simulink model "DinamicaCinematicaControleAtitude"  (R2024a)
settings: Solver=FixedStepAuto  StartTime=0.0  StopTime=tf  FixedStep=step_modelo  RelTol=1e-3
values from neighbouring files (symbols this model uses):
  mi = 3.9860044189*10^14    (= 398600441890000)    [constantes.m]
undefined symbols (not defined in the file or in its folder): a0_ini, AttKd_x, AttKd_y, AttKd_z, AttKp_x, AttKp_y, AttKp_z, e0_ini, f0_ini, giro, giro_bias, giro_ruido, Ixx, Iyy, Izz, omega0_ini, omega1_rel_ini, omega2_rel_ini, omega3_rel_ini, phi_i, psi_i, theta_i
libraries: dspsrcs4 x3, matrix_library x2, sharedutil x2, aerolibutil x1
settings Model: Creator=rodri  LastModifiedBy=rodri
settings DataIOCC: SaveOutput=off  SaveTime=off
settings RTWCC: GPUComputeCapability=3.5

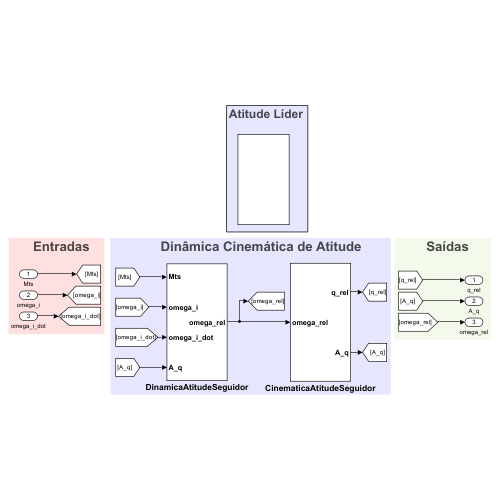
[thumbnail: Simulink's stored preview of the top-level diagram]
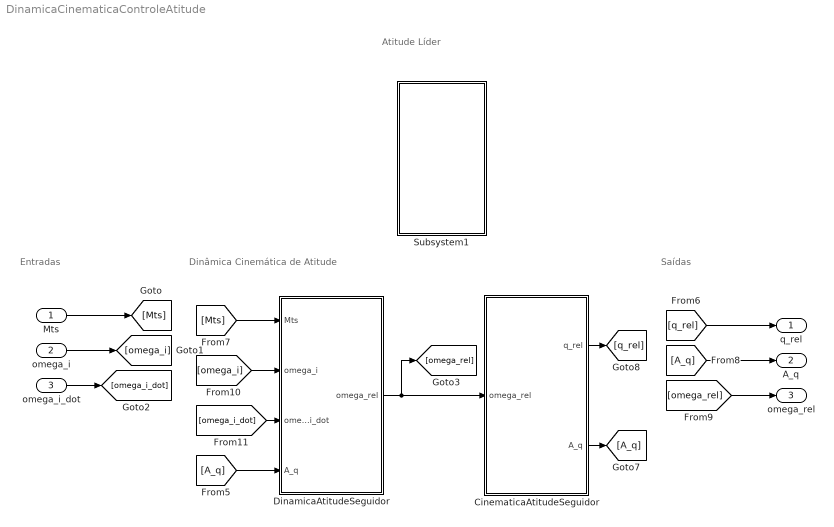
== system DinamicaCinematicaControleAtitude ==
  note: Dinâmica Cinemática de Atitude
  note: Entradas
  note: Saídas
  note: Atitude Líder
  Mts : Inport  OutDataTypeStr=double  PortDimensions=[3,1]
  omega_i : Inport  Port=2  OutDataTypeStr=double
  omega_i_dot : Inport  Port=3  OutDataTypeStr=double  PortDimensions=[3,1]
  CinematicaAtitudeSeguidor : Subsystem
  DinamicaAtitudeSeguidor : Subsystem
  Subsystem1 : Subsystem
  q_rel : Outport
  A_q : Outport  Port=2  PortDimensions=[3,3]
  omega_rel : Outport  Port=3
  wires:
  DinamicaAtitudeSeguidor/1(omega_rel) -> [omega_rel], CinematicaAtitudeSeguidor/1(omega_rel)
  CinematicaAtitudeSeguidor/2(A_q) -> [A_q]
  CinematicaAtitudeSeguidor/1(q_rel) -> [q_rel]
  omega_i/1 -> [omega_i]
  omega_i_dot/1 -> [omega_i_dot]
  [A_q] -> DinamicaAtitudeSeguidor/4(A_q)
  [Mts] -> DinamicaAtitudeSeguidor/1(Mts)
  [omega_i] -> DinamicaAtitudeSeguidor/2(omega_i)
  [omega_i_dot] -> DinamicaAtitudeSeguidor/3(omega_i_dot)
  [q_rel] -> q_rel/1
  [A_q] -> A_q/1
  [omega_rel] -> omega_rel/1
  Mts/1 -> [Mts]

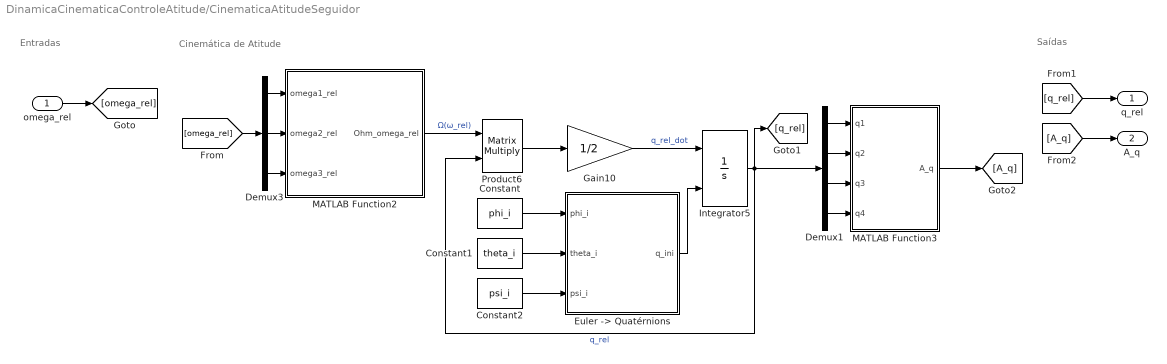
== system DinamicaCinematicaControleAtitude/CinematicaAtitudeSeguidor ==
  note: Cinemática de Atitude
  note: Entradas
  note: Saídas
  omega_rel : Inport
  Constant : Constant  Value=phi_i  SampleTime=-1
  Constant1 : Constant  Value=theta_i  SampleTime=-1
  Constant2 : Constant  Value=psi_i  SampleTime=-1
  Demux1 : Demux
  Demux3 : Demux  Outputs=3
  "Euler -> Quatérnions" : MATLAB Function  TreatAsAtomicUnit=on
  Gain10 : Gain  Gain=1/2
  Integrator5 : Integrator  InitialConditionSource=external  InitialCondition=[1; 0; 0; 0]
  MATLAB Function2 : MATLAB Function  TreatAsAtomicUnit=on
  MATLAB Function3 : MATLAB Function  TreatAsAtomicUnit=on
  Product6 : Product  Multiplication=Matrix(*)
  q_rel : Outport
  A_q : Outport  Port=2  PortDimensions=[3,3]
  wires:
  "Euler -> Quatérnions"/1(q_ini) -> Integrator5/2
  Demux1/2 -> MATLAB Function3/2(q2)
  Demux3/1 -> MATLAB Function2/1(omega1_rel)
  MATLAB Function2/1(Ohm_omega_rel) -> Product6/1  "Ω(ω_rel)"
  Demux1/4 -> MATLAB Function3/4(q4)
  Demux3/3 -> MATLAB Function2/3(omega3_rel)
  Demux3/2 -> MATLAB Function2/2(omega2_rel)
  Integrator5/1 -> Product6/2, Demux1/1, [q_rel]  "q_rel"
  Demux1/3 -> MATLAB Function3/3(q3)
  Gain10/1 -> Integrator5/1  "q_rel_dot"
  Demux1/1 -> MATLAB Function3/1(q1)
  Product6/1 -> Gain10/1
  [omega_rel] -> Demux3/1
  omega_rel/1 -> [omega_rel]
  [q_rel] -> q_rel/1
  [A_q] -> A_q/1
  MATLAB Function3/1(A_q) -> [A_q]
  Constant/1 -> "Euler -> Quatérnions"/1(phi_i)
  Constant1/1 -> "Euler -> Quatérnions"/2(theta_i)
  Constant2/1 -> "Euler -> Quatérnions"/3(psi_i)

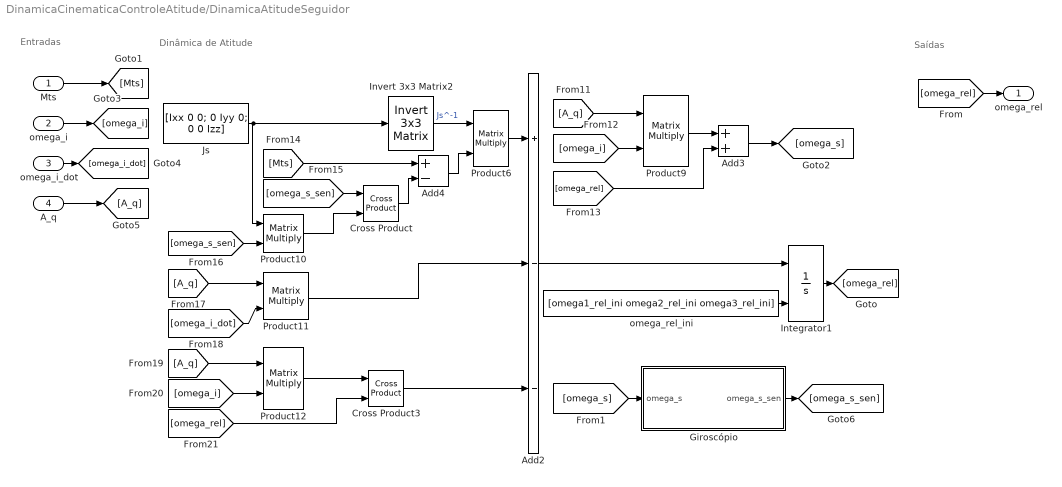
== system DinamicaCinematicaControleAtitude/DinamicaAtitudeSeguidor ==
  note: Dinâmica de Atitude
  note: Saídas
  note: Entradas
  Mts : Inport
  omega_i : Inport  Port=2
  omega_i_dot : Inport  Port=3
  A_q : Inport  Port=4
  Add2 : Sum  Inputs=+--
  Add3 : Sum
  Add4 : Sum  Inputs=+-
  Cross Product : matrix_library/Cross Product
  Cross Product3 : matrix_library/Cross Product
  Giroscópio : Subsystem
  Integrator1 : Integrator  InitialConditionSource=external  InitialCondition=[0; 0; 0]
  Invert 3x3 Matrix2 : aerolibutil/Invert  3x3 Matrix
  Js : Constant  Value=[Ixx 0 0; 0 Iyy 0; 0 0 Izz]
  Product{6,9..12} (5 alike) : Product  Multiplication=Matrix(*)
  omega_rel_ini : Constant  Value=[omega1_rel_ini omega2_rel_ini omega3_rel_ini]
  omega_rel : Outport
  wires:
  Integrator1/1 -> [omega_rel]
  Add2/1 -> Integrator1/1
  Invert 3x3 Matrix2/1 -> Product6/1  "Js^-1"
  omega_rel_ini/1 -> Integrator1/2
  [A_q] -> Product9/1
  [omega_i] -> Product9/2
  Product9/1 -> Add3/1
  [omega_rel] -> Add3/2
  Add3/1 -> [omega_s]
  [Mts] -> Add4/1
  Cross Product/1 -> Add4/2
  [omega_s_sen] -> Cross Product/1
  Js/1 -> Product10/1, Invert 3x3 Matrix2/1
  [omega_s_sen] -> Product10/2
  Product10/1 -> Cross Product/2
  Add4/1 -> Product6/2
  Product6/1 -> Add2/1
  [A_q] -> Product11/1
  [omega_i_dot] -> Product11/2
  Product11/1 -> Add2/2
  [A_q] -> Product12/1
  [omega_i] -> Product12/2
  Product12/1 -> Cross Product3/1
  [omega_rel] -> Cross Product3/2
  Cross Product3/1 -> Add2/3
  omega_i/1 -> [omega_i]
  A_q/1 -> [A_q]
  [omega_rel] -> omega_rel/1
  Mts/1 -> [Mts]
  omega_i_dot/1 -> [omega_i_dot]
  [omega_s] -> Giroscópio/1(omega_s)
  Giroscópio/1(omega_s_sen) -> [omega_s_sen]

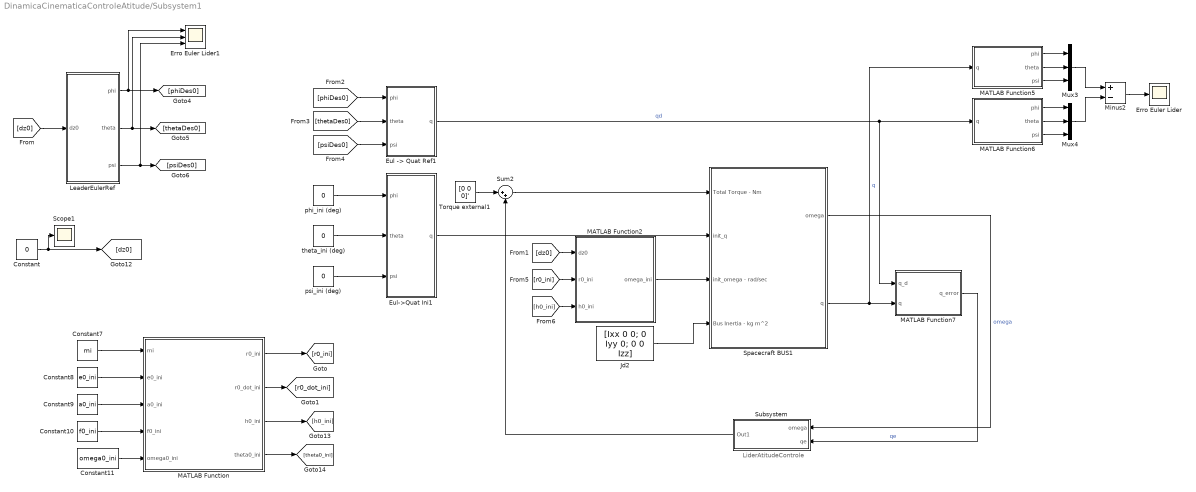
== system DinamicaCinematicaControleAtitude/Subsystem1 ==
  note: LiderAtitudeControle
  Constant : Constant  Value=0
  Constant10 : Constant  Value=f0_ini
  Constant11 : Constant  Value=omega0_ini
  Constant7 : Constant  Value=mi
  Constant8 : Constant  Value=e0_ini
  Constant9 : Constant  Value=a0_ini
  Erro Euler Lider : Scope
  Erro Euler Lider1 : Scope  NumInputPorts=3
  "Eul -> Quat Ref1" : MATLAB Function  TreatAsAtomicUnit=on
  Eul->Quat Ini1 : MATLAB Function  TreatAsAtomicUnit=on
  Jd2 : Constant  Value=[Ixx 0 0; 0 Iyy 0; 0 0 Izz]
  LeaderEulerRef : Subsystem
  MATLAB Function : MATLAB Function  TreatAsAtomicUnit=on
  MATLAB Function2 : MATLAB Function  TreatAsAtomicUnit=on
  MATLAB Function5 : MATLAB Function  TreatAsAtomicUnit=on
  MATLAB Function6 : MATLAB Function  TreatAsAtomicUnit=on
  MATLAB Function7 : MATLAB Function  TreatAsAtomicUnit=on
  Minus2 : Sum  Inputs=+-
  Mux3 : Mux  Inputs=3
  Mux4 : Mux  Inputs=3
  Scope1 : Scope
  Spacecraft BUS1 : Subsystem
  Subsystem : Subsystem
  Sum2 : Sum  Inputs=|++
  Torque external1 : Constant  Value=[0 0 0]'
  phi_ini (deg) : Constant  Value=0
  psi_ini (deg) : Constant  Value=0
  theta_ini (deg) : Constant  Value=0
  wires:
  "Eul -> Quat Ref1"/1(q) -> MATLAB Function7/1(q_d), MATLAB Function6/1(q)  "qd"
  LeaderEulerRef/3(psi) -> Erro Euler Lider1/3, [psiDes0]
  Spacecraft BUS1/2(q) -> MATLAB Function5/1(q), MATLAB Function7/2(q)  "q"
  MATLAB Function5/3(psi) -> Mux3/3
  [phiDes0] -> "Eul -> Quat Ref1"/1(phi)
  MATLAB Function5/2(theta) -> Mux3/2
  MATLAB Function6/1(phi) -> Mux4/1
  MATLAB Function5/1(phi) -> Mux3/1
  [r0_ini] -> MATLAB Function2/2(r0_ini)
  [thetaDes0] -> "Eul -> Quat Ref1"/2(theta)
  Torque external1/1 -> Sum2/1
  MATLAB Function6/3(psi) -> Mux4/3
  [h0_ini] -> MATLAB Function2/3(h0_ini)
  [dz0] -> LeaderEulerRef/1(dz0)
  Mux3/1 -> Minus2/1
  Minus2/1 -> Erro Euler Lider/1
  theta_ini (deg)/1 -> Eul->Quat Ini1/2(theta)
  LeaderEulerRef/1(phi) -> Erro Euler Lider1/1, [phiDes0]
  Jd2/1 -> Spacecraft BUS1/4(Bus Inertia - kg m^2)
  Sum2/1 -> Spacecraft BUS1/1(Total Torque - Nm)
  Eul->Quat Ini1/1(q) -> Spacecraft BUS1/2(init_q)
  LeaderEulerRef/2(theta) -> Erro Euler Lider1/2, [thetaDes0]
  Mux4/1 -> Minus2/2
  [psiDes0] -> "Eul -> Quat Ref1"/3(psi)
  Constant/1 -> Scope1/1, [dz0]
  Subsystem/1(Out1) -> Sum2/2
  [dz0] -> MATLAB Function2/1(dz0)
  psi_ini (deg)/1 -> Eul->Quat Ini1/3(psi)
  phi_ini (deg)/1 -> Eul->Quat Ini1/1(phi)
  MATLAB Function7/1(q_error) -> Subsystem/2(qe)  "qe"
  Spacecraft BUS1/1(omega) -> Subsystem/1(omega)  "omega"
  MATLAB Function2/1(omega_ini) -> Spacecraft BUS1/3(init_omega - rad/sec)
  MATLAB Function6/2(theta) -> Mux4/2
  MATLAB Function/3(h0_ini) -> [h0_ini]
  Constant10/1 -> MATLAB Function/4(f0_ini)
  Constant11/1 -> MATLAB Function/5(omega0_ini)
  MATLAB Function/1(r0_ini) -> [r0_ini]
  Constant7/1 -> MATLAB Function/1(mi)
  Constant8/1 -> MATLAB Function/2(e0_ini)
  Constant9/1 -> MATLAB Function/3(a0_ini)
  MATLAB Function/4(theta0_ini) -> [theta0_ini]
  MATLAB Function/2(r0_dot_ini) -> [r0_dot_ini]

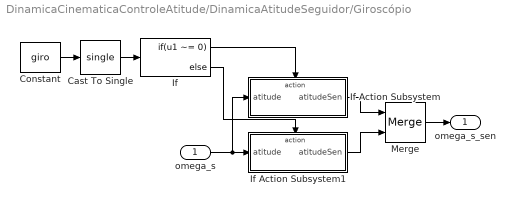
== system DinamicaCinematicaControleAtitude/DinamicaAtitudeSeguidor/Giroscópio ==
  omega_s : Inport
  Cast To Single : DataTypeConversion  OutDataTypeStr=single  SaturateOnIntegerOverflow=off  RndMeth=Floor
  Constant : Constant  Value=giro
  If : If  IfExpression=u1 ~= 0
  If Action Subsystem : Subsystem  TreatAsAtomicUnit=on
  If Action Subsystem1 : Subsystem  TreatAsAtomicUnit=on
  Merge : Merge
  omega_s_sen : Outport
  wires:
  Cast To Single/1 -> If/1
  If/2 -> If Action Subsystem1/Action
  If Action Subsystem/1(atitudeSen) -> Merge/1
  If/1 -> If Action Subsystem/Action
  Merge/1 -> omega_s_sen/1
  Constant/1 -> Cast To Single/1
  If Action Subsystem1/1(atitudeSen) -> Merge/2
  omega_s/1 -> If Action Subsystem/1(atitude), If Action Subsystem1/1(atitude)

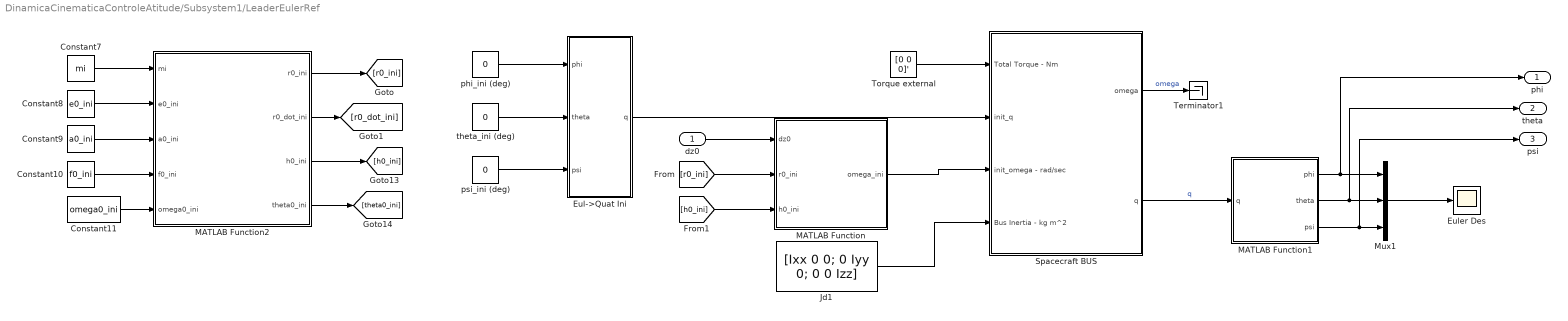
== system DinamicaCinematicaControleAtitude/Subsystem1/LeaderEulerRef ==
  dz0 : Inport
  Constant10 : Constant  Value=f0_ini
  Constant11 : Constant  Value=omega0_ini
  Constant7 : Constant  Value=mi
  Constant8 : Constant  Value=e0_ini
  Constant9 : Constant  Value=a0_ini
  Eul->Quat Ini : MATLAB Function  TreatAsAtomicUnit=on
  Euler Des : Scope
  Jd1 : Constant  Value=[Ixx 0 0; 0 Iyy 0; 0 0 Izz]
  MATLAB Function : MATLAB Function  TreatAsAtomicUnit=on
  MATLAB Function1 : MATLAB Function  TreatAsAtomicUnit=on
  MATLAB Function2 : MATLAB Function  TreatAsAtomicUnit=on
  Mux1 : Mux  Inputs=3
  Spacecraft BUS : Subsystem
  Terminator1 : Terminator
  Torque external : Constant  Value=[0 0 0]'
  phi_ini (deg) : Constant  Value=0
  psi_ini (deg) : Constant  Value=0
  theta_ini (deg) : Constant  Value=0
  phi : Outport
  theta : Outport  Port=2
  psi : Outport  Port=3
  wires:
  MATLAB Function1/2(theta) -> theta/1, Mux1/2
  [r0_ini] -> MATLAB Function/2(r0_ini)
  MATLAB Function1/3(psi) -> psi/1, Mux1/3
  MATLAB Function/1(omega_ini) -> Spacecraft BUS/3(init_omega - rad/sec)
  MATLAB Function1/1(phi) -> phi/1, Mux1/1
  psi_ini (deg)/1 -> Eul->Quat Ini/3(psi)
  Spacecraft BUS/2(q) -> MATLAB Function1/1(q)  "q"
  dz0/1 -> MATLAB Function/1(dz0)
  Mux1/1 -> Euler Des/1
  Eul->Quat Ini/1(q) -> Spacecraft BUS/2(init_q)
  theta_ini (deg)/1 -> Eul->Quat Ini/2(theta)
  Spacecraft BUS/1(omega) -> Terminator1/1  "omega"
  [h0_ini] -> MATLAB Function/3(h0_ini)
  phi_ini (deg)/1 -> Eul->Quat Ini/1(phi)
  Torque external/1 -> Spacecraft BUS/1(Total Torque - Nm)
  Jd1/1 -> Spacecraft BUS/4(Bus Inertia - kg m^2)
  MATLAB Function2/2(r0_dot_ini) -> [r0_dot_ini]
  Constant10/1 -> MATLAB Function2/4(f0_ini)
  MATLAB Function2/3(h0_ini) -> [h0_ini]
  Constant7/1 -> MATLAB Function2/1(mi)
  Constant9/1 -> MATLAB Function2/3(a0_ini)
  Constant8/1 -> MATLAB Function2/2(e0_ini)
  Constant11/1 -> MATLAB Function2/5(omega0_ini)
  MATLAB Function2/1(r0_ini) -> [r0_ini]
  MATLAB Function2/4(theta0_ini) -> [theta0_ini]

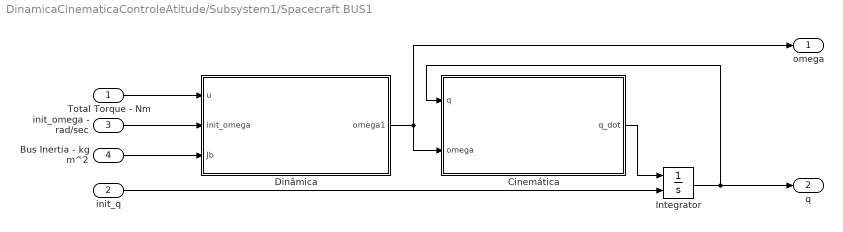
== system DinamicaCinematicaControleAtitude/Subsystem1/Spacecraft BUS1 ==
  Total Torque - Nm : Inport
  init_q : Inport  Port=2
  init_omega - rad/sec : Inport  Port=3
  Bus Inertia - kg m^2 : Inport  Port=4
  Cinemática : Subsystem
  Dinâmica : Subsystem
  Integrator : Integrator  InitialConditionSource=external
  omega : Outport  VectorParamsAs1DForOutWhenUnconnected=off
  q : Outport  Port=2  VectorParamsAs1DForOutWhenUnconnected=off
  wires:
  Bus Inertia - kg m^2/1 -> Dinâmica/3(Jb)
  Dinâmica/1(omega1) -> omega/1, Cinemática/2(omega)
  init_q/1 -> Integrator/2
  init_omega - rad/sec/1 -> Dinâmica/2(init_omega)
  Total Torque - Nm/1 -> Dinâmica/1(u)
  Integrator/1 -> q/1, Cinemática/1(q)
  Cinemática/1(q_dot) -> Integrator/1

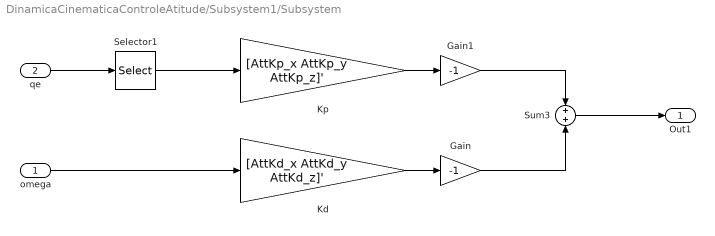
== system DinamicaCinematicaControleAtitude/Subsystem1/Subsystem ==
  omega : Inport
  qe : Inport  Port=2
  Gain : Gain  Gain=-1
  Gain1 : Gain  Gain=-1
  Kd : Gain  Gain=[AttKd_x AttKd_y AttKd_z]'
  Kp : Gain  Gain=[AttKp_x AttKp_y AttKp_z]'
  Selector1 : Selector  InputPortWidth=4  IndexOptions=Index vector (dialog)  Indices=[1 2 3 ]  OutputSizes=1
  Sum3 : Sum  Inputs=+|+
  Out1 : Outport
  wires:
  Kp/1 -> Gain1/1
  Selector1/1 -> Kp/1
  Kd/1 -> Gain/1
  qe/1 -> Selector1/1
  Sum3/1 -> Out1/1
  omega/1 -> Kd/1
  Gain/1 -> Sum3/2
  Gain1/1 -> Sum3/1

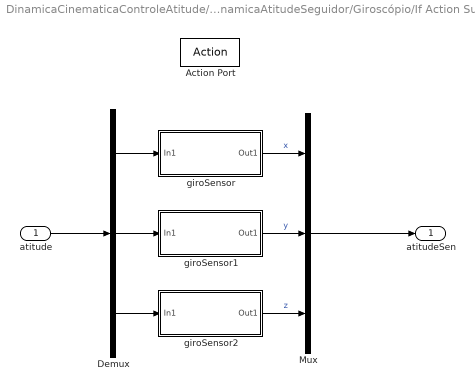
== system DinamicaCinematicaControleAtitude/DinamicaAtitudeSeguidor/Giroscópio/If Action Subsystem ==
  atitude : Inport
  Action Port : ActionPort  ActionPortLabel=if(u1 ~= 0)
  Demux : Demux  Outputs=3
  Mux : Mux  Inputs=3
  giroSensor : Subsystem
  giroSensor1 : Subsystem
  giroSensor2 : Subsystem
  atitudeSen : Outport
  wires:
  Demux/3 -> giroSensor2/1(In1)
  Demux/2 -> giroSensor1/1(In1)
  Demux/1 -> giroSensor/1(In1)
  atitude/1 -> Demux/1
  giroSensor/1(Out1) -> Mux/1  "x"
  giroSensor1/1(Out1) -> Mux/2  "y"
  giroSensor2/1(Out1) -> Mux/3  "z"
  Mux/1 -> atitudeSen/1

== system DinamicaCinematicaControleAtitude/DinamicaAtitudeSeguidor/Giroscópio/If Action Subsystem1 ==
  atitude : Inport
  Action Port : ActionPort  ActionPortLabel=else
  atitudeSen : Outport
  wires:
  atitude/1 -> atitudeSen/1

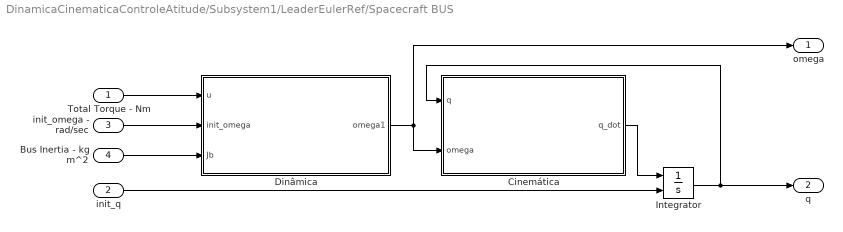
== system DinamicaCinematicaControleAtitude/Subsystem1/LeaderEulerRef/Spacecraft BUS ==
  Total Torque - Nm : Inport
  init_q : Inport  Port=2
  init_omega - rad/sec : Inport  Port=3
  Bus Inertia - kg m^2 : Inport  Port=4
  Cinemática : Subsystem
  Dinâmica : Subsystem
  Integrator : Integrator  InitialConditionSource=external
  omega : Outport  VectorParamsAs1DForOutWhenUnconnected=off
  q : Outport  Port=2  VectorParamsAs1DForOutWhenUnconnected=off
  wires:
  Bus Inertia - kg m^2/1 -> Dinâmica/3(Jb)
  Dinâmica/1(omega1) -> omega/1, Cinemática/2(omega)
  init_q/1 -> Integrator/2
  init_omega - rad/sec/1 -> Dinâmica/2(init_omega)
  Total Torque - Nm/1 -> Dinâmica/1(u)
  Integrator/1 -> q/1, Cinemática/1(q)
  Cinemática/1(q_dot) -> Integrator/1

== system DinamicaCinematicaControleAtitude/Subsystem1/Spacecraft BUS1/Cinemática ==
  q : Inport
  omega : Inport  Port=2
  MATLAB Function : MATLAB Function  TreatAsAtomicUnit=on
  q_dot : Outport  VectorParamsAs1DForOutWhenUnconnected=off
  wires:
  q/1 -> MATLAB Function/2(q)
  omega/1 -> MATLAB Function/1(omega)
  MATLAB Function/1(q_dot) -> q_dot/1

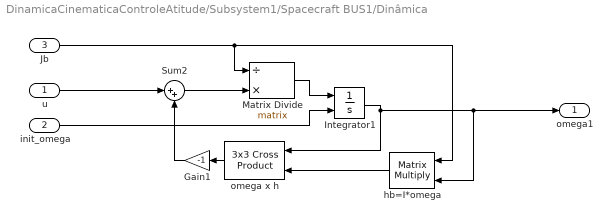
== system DinamicaCinematicaControleAtitude/Subsystem1/Spacecraft BUS1/Dinâmica ==
  u : Inport
  init_omega : Inport  Port=2
  Jb : Inport  Port=3
  Gain1 : Gain  Gain=-1
  Integrator1 : Integrator  InitialConditionSource=external  ZeroCross=off
  Matrix Divide : Product  Inputs=/*  Multiplication=Matrix(*)
  Sum2 : Sum  Inputs=|++
  hb=I*omega : Product  Multiplication=Matrix(*)
  omega x h : sharedutil/3x3 Cross Product  aMode=aMode
  omega1 : Outport  VectorParamsAs1DForOutWhenUnconnected=off
  wires:
  Jb/1 -> hb=I*omega/1, Matrix Divide/1
  Matrix Divide/1 -> Integrator1/1
  u/1 -> Sum2/1
  omega x h/1 -> Gain1/1
  hb=I*omega/1 -> omega x h/2
  Sum2/1 -> Matrix Divide/2
  init_omega/1 -> Integrator1/2
  Integrator1/1 -> hb=I*omega/2, omega1/1, omega x h/1
  Gain1/1 -> Sum2/2

== system DinamicaCinematicaControleAtitude/DinamicaAtitudeSeguidor/Giroscópio/If Action Subsystem/giroSensor ==
  In1 : Inport
  Add1 : Sum
  Add2 : Sum
  Constant : Constant  Value=deg2rad(giro_bias)
  Random Source1 : dspsrcs4/Random Source  SrcType=Uniform  MinVal=-deg2rad(giro_ruido)  MaxVal=deg2rad(giro_ruido)  MeanVal=0  VarVal=1  RepMode=Not repeatable  rawSeed=1  IsInherit=off  SampTime=step_modelo  SampFrame=1  OutComplex=Real  DataType=double  SimulateUsing=Code generation
  Out1 : Outport
  wires:
  Random Source1/1 -> Add2/1
  In1/1 -> Add1/2
  Constant/1 -> Add1/1
  Add1/1 -> Add2/2
  Add2/1 -> Out1/1

== system DinamicaCinematicaControleAtitude/DinamicaAtitudeSeguidor/Giroscópio/If Action Subsystem/giroSensor1 ==
  In1 : Inport
  Add1 : Sum
  Add2 : Sum
  Constant : Constant  Value=deg2rad(giro_bias)
  Random Source1 : dspsrcs4/Random Source  SrcType=Uniform  MinVal=-deg2rad(giro_ruido)  MaxVal=deg2rad(giro_ruido)  MeanVal=0  VarVal=1  RepMode=Not repeatable  rawSeed=1  IsInherit=off  SampTime=step_modelo  SampFrame=1  OutComplex=Real  DataType=double  SimulateUsing=Code generation
  Out1 : Outport
  wires:
  Random Source1/1 -> Add2/1
  Add2/1 -> Out1/1
  In1/1 -> Add1/2
  Constant/1 -> Add1/1
  Add1/1 -> Add2/2

== system DinamicaCinematicaControleAtitude/DinamicaAtitudeSeguidor/Giroscópio/If Action Subsystem/giroSensor2 ==
  In1 : Inport
  Add1 : Sum
  Add2 : Sum
  Constant : Constant  Value=deg2rad(giro_bias)
  Random Source1 : dspsrcs4/Random Source  SrcType=Uniform  MinVal=-deg2rad(giro_ruido)  MaxVal=deg2rad(giro_ruido)  MeanVal=0  VarVal=1  RepMode=Not repeatable  rawSeed=1  IsInherit=off  SampTime=step_modelo  SampFrame=1  OutComplex=Real  DataType=double  SimulateUsing=Code generation
  Out1 : Outport
  wires:
  Random Source1/1 -> Add2/1
  Add2/1 -> Out1/1
  In1/1 -> Add1/2
  Constant/1 -> Add1/1
  Add1/1 -> Add2/2

== system DinamicaCinematicaControleAtitude/Subsystem1/LeaderEulerRef/Spacecraft BUS/Cinemática ==
  q : Inport
  omega : Inport  Port=2
  MATLAB Function : MATLAB Function  TreatAsAtomicUnit=on
  q_dot : Outport  VectorParamsAs1DForOutWhenUnconnected=off
  wires:
  q/1 -> MATLAB Function/2(q)
  omega/1 -> MATLAB Function/1(omega)
  MATLAB Function/1(q_dot) -> q_dot/1

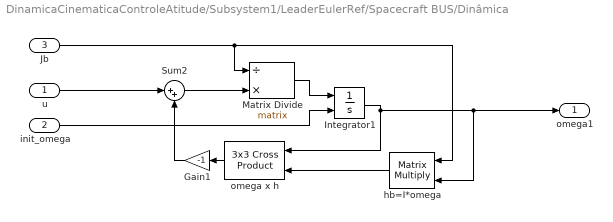
== system DinamicaCinematicaControleAtitude/Subsystem1/LeaderEulerRef/Spacecraft BUS/Dinâmica ==
  u : Inport
  init_omega : Inport  Port=2
  Jb : Inport  Port=3
  Gain1 : Gain  Gain=-1
  Integrator1 : Integrator  InitialConditionSource=external  ZeroCross=off
  Matrix Divide : Product  Inputs=/*  Multiplication=Matrix(*)
  Sum2 : Sum  Inputs=|++
  hb=I*omega : Product  Multiplication=Matrix(*)
  omega x h : sharedutil/3x3 Cross Product  aMode=aMode
  omega1 : Outport  VectorParamsAs1DForOutWhenUnconnected=off
  wires:
  Jb/1 -> hb=I*omega/1, Matrix Divide/1
  Matrix Divide/1 -> Integrator1/1
  u/1 -> Sum2/1
  omega x h/1 -> Gain1/1
  hb=I*omega/1 -> omega x h/2
  Sum2/1 -> Matrix Divide/2
  init_omega/1 -> Integrator1/2
  Integrator1/1 -> hb=I*omega/2, omega1/1, omega x h/1
  Gain1/1 -> Sum2/2

== matlab function DinamicaCinematicaControleAtitude/Subsystem1/MATLAB Function2 ==
  data: dz0 input; omega_ini output; r0_ini input; h0_ini input
function omega_ini = fcn(dz0,r0_ini,h0_ini)

omega_x_ini = dz0*r0_ini/h0_ini;
omega_y_ini = 0;
omega_z_ini = h0_ini/(r0_ini^2);

omega_ini = [omega_x_ini omega_y_ini omega_z_ini]';

== matlab function DinamicaCinematicaControleAtitude/Subsystem1/MATLAB Function5 ==
  data: q input; phi output; theta output; psi output
function [phi,theta,psi] = fcn(q)

q1 = q(1);
q2 = q(2);
q3 = q(3);
q4 = q(4);

eul = quat2eul([q1 q2 q3 q4]);

phi = rad2deg(eul(1));
theta = rad2deg(eul(2));
psi = rad2deg(eul(3));

== matlab function DinamicaCinematicaControleAtitude/Subsystem1/MATLAB Function6 ==
  data: q input; phi output; theta output; psi output
function [phi,theta,psi] = fcn(q)

q1 = q(1);
q2 = q(2);
q3 = q(3);
q4 = q(4);

eul = quat2eul([q1 q2 q3 q4]);

phi = rad2deg(eul(1));
theta = rad2deg(eul(2));
psi = rad2deg(eul(3));

== matlab function DinamicaCinematicaControleAtitude/Subsystem1/MATLAB Function7 ==
  data: q_d input; q_error output; q input
function q_error = fcn(q_d,q)

qt1 = q_d(1);
qt2 = q_d(2);
qt3 = q_d(3);
qt4 = q_d(4);

qs1 = q(1);
qs2 = q(2);
qs3 = q(3);
qs4 = q(4);

q_error = [qt4 qt3 -qt2 -qt1
    -qt3 qt4 qt1 -qt2
    qt2 -qt1 qt4 -qt3
    qt1 qt2 qt3 qt4]*[qs1;qs2;qs3;qs4];

== matlab function DinamicaCinematicaControleAtitude/Subsystem1/Spacecraft BUS1/Cinemática/MATLAB Function ==
  data: omega input; q_dot output; q input
function q_dot = fcn(omega,q)

omegax = omega(1);
omegay = omega(2);
omegaz = omega(3);


Ohm = [0 omegaz -omegay omegax
    -omegaz 0 omegax omegay
    omegay -omegax 0 omegaz
    -omegax -omegay -omegaz 0];

q_dot = (1/2)*Ohm*q;

== matlab function DinamicaCinematicaControleAtitude/Subsystem1/LeaderEulerRef/Eul->Quat Ini ==
  data: phi input; q output; theta input; psi input
function q = fcn(phi,theta,psi)

q = eul2quat(deg2rad([phi theta psi]))';

== matlab function DinamicaCinematicaControleAtitude/CinematicaAtitudeSeguidor/MATLAB Function3 ==
  data: q1 input; A_q output; q2 input; q3 input; q4 input
function A_q = fcn(q1,q2,q3,q4)

A_q_11 = q1^2-q2^2-q3^2+q4^2;
A_q_12 = 2*(q1*q2+q3*q4);
A_q_13 = 2*(q1*q3-q2*q4);
A_q_21 = 2*(q1*q2-q3*q4);
A_q_22 = -q1^2+q2^2-q3^2+q4^2;
A_q_23 = 2*(q2*q3+q1*q4);
A_q_31 = 2*(q1*q3+q2*q4);
A_q_32 = 2*(q2*q3-q1*q4);
A_q_33 = -q1^2-q2^2+q3^2+q4^2;

A_q = [A_q_11, A_q_12, A_q_13;
       A_q_21, A_q_22, A_q_23;
       A_q_31, A_q_32, A_q_33];

== matlab function DinamicaCinematicaControleAtitude/CinematicaAtitudeSeguidor/Euler -> Quatérnions ==
  data: phi_i input; q_ini output; theta_i input; psi_i input
function q_ini = fcn(phi_i,theta_i,psi_i)

q_ref = eul2quat([phi_i theta_i psi_i]);

q_ini = [q_ref(2),q_ref(3),q_ref(4),q_ref(1)]';

== matlab function DinamicaCinematicaControleAtitude/Subsystem1/LeaderEulerRef/MATLAB Function2 ==
  data: mi input; r0_ini output; e0_ini input; a0_ini input; f0_ini input; r0_dot_ini output; h0_ini output; omega0_ini input; theta0_ini output
function [r0_ini,r0_dot_ini,h0_ini,theta0_ini] = fcn(mi,e0_ini,a0_ini,f0_ini,omega0_ini)

r0_ini = a0_ini*(1 - e0_ini^2)/(1 + e0_ini*cos(f0_ini));
r0_dot_ini = e0_ini*sin(f0_ini)*sqrt(mi/(a0_ini*(1 - e0_ini^2)));
h0_ini = sqrt(-(e0_ini^2 - 1)*mi*a0_ini);
theta0_ini = omega0_ini + f0_ini;

== matlab function DinamicaCinematicaControleAtitude/Subsystem1/LeaderEulerRef/MATLAB Function1 ==
  data: q input; phi output; theta output; psi output
function [phi,theta,psi] = fcn(q)

q1 = q(1);
q2 = q(2);
q3 = q(3);
q4 = q(4);

eul = quat2eul([q1 q2 q3 q4]);

phi = rad2deg((eul(1)));
theta = rad2deg((eul(2)));
psi = rad2deg((eul(3)));

== matlab function DinamicaCinematicaControleAtitude/CinematicaAtitudeSeguidor/MATLAB Function2 ==
  data: omega1_rel input; Ohm_omega_rel output; omega2_rel input; omega3_rel input
function Ohm_omega_rel  = fcn(omega1_rel,omega2_rel,omega3_rel)

Ohm_omega_rel = [0 omega3_rel -omega2_rel omega1_rel
    -omega3_rel 0 omega1_rel omega2_rel
    omega2_rel -omega1_rel 0 omega3_rel
    -omega1_rel -omega2_rel -omega3_rel 0];

== matlab function DinamicaCinematicaControleAtitude/Subsystem1/MATLAB Function ==
  data: mi input; r0_ini output; e0_ini input; a0_ini input; f0_ini input; r0_dot_ini output; h0_ini output; omega0_ini input; theta0_ini output
function [r0_ini,r0_dot_ini,h0_ini,theta0_ini] = fcn(mi,e0_ini,a0_ini,f0_ini,omega0_ini)

r0_ini = a0_ini*(1 - e0_ini^2)/(1 + e0_ini*cos(f0_ini));
r0_dot_ini = e0_ini*sin(f0_ini)*sqrt(mi/(a0_ini*(1 - e0_ini^2)));
h0_ini = sqrt(-(e0_ini^2 - 1)*mi*a0_ini);
theta0_ini = omega0_ini + f0_ini;

== matlab function DinamicaCinematicaControleAtitude/Subsystem1/LeaderEulerRef/Spacecraft BUS/Cinemática/MATLAB Function ==
  data: omega input; q_dot output; q input
function q_dot = fcn(omega,q)

omegax = omega(1);
omegay = omega(2);
omegaz = omega(3);


Ohm = [0 omegaz -omegay omegax
    -omegaz 0 omegax omegay
    omegay -omegax 0 omegaz
    -omegax -omegay -omegaz 0];

q_dot = (1/2)*Ohm*q;

== matlab function DinamicaCinematicaControleAtitude/Subsystem1/LeaderEulerRef/MATLAB Function ==
  data: dz0 input; omega_ini output; r0_ini input; h0_ini input
function omega_ini = fcn(dz0,r0_ini,h0_ini)

omega_x_ini = dz0*r0_ini/h0_ini;
omega_y_ini = 0;
omega_z_ini = h0_ini/(r0_ini^2);

omega_ini = [omega_x_ini omega_y_ini omega_z_ini]';

== matlab function DinamicaCinematicaControleAtitude/Subsystem1/Eul -> Quat Ref1 ==
  data: phi input; q output; theta input; psi input
function q = fcn(phi,theta,psi)

q = eul2quat(deg2rad([phi theta psi]))';

== matlab function DinamicaCinematicaControleAtitude/Subsystem1/Eul->Quat Ini1 ==
  data: phi input; q output; theta input; psi input
function q = fcn(phi,theta,psi)

q = eul2quat(deg2rad([phi theta psi]))';
